simulink model "Simulink_v4"  (R2023b)
settings: Solver=FixedStepDiscrete  StartTime=0.0  StopTime=100  FixedStep=0.01  RelTol=1e-3
settings Model: PacingRate=10  Creator=MrLove  LastModifiedBy=MrLove

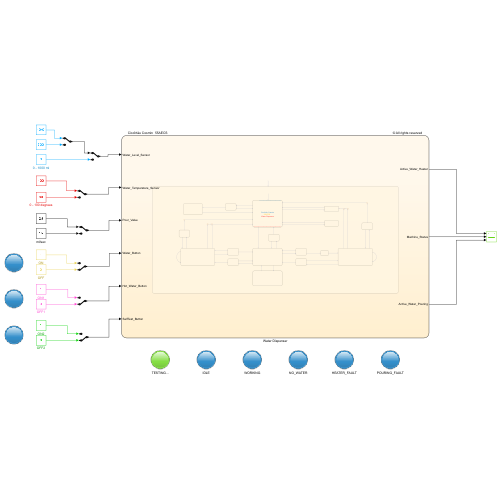
[thumbnail: Simulink's stored preview of the top-level diagram]
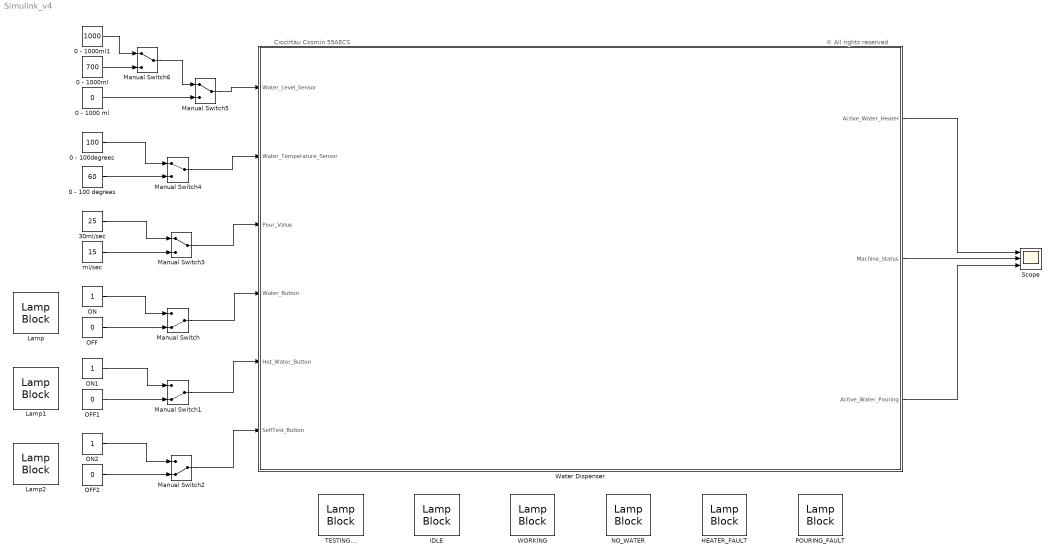
== system Simulink_v4 ==
  note: © All rights reserved
  note: Ciocîrtău Cosmin 55AECS
  0 - 100 degrees : Constant  Value=60
  0 - 1000 ml : Constant  Value=0
  0 - 1000ml : Constant  Value=700
  0 - 1000ml1 : Constant  Value=1000
  0 - 100degrees : Constant  Value=100
  30ml/sec : Constant  Value=25
  HEATER_FAULT : LampBlock  LabelPosition=Hide
  IDLE : LampBlock  LabelPosition=Hide
  Lamp : LampBlock  LabelPosition=Hide
  Lamp1 : LampBlock  LabelPosition=Hide
  Lamp2 : LampBlock  LabelPosition=Hide
  Manual Switch : ManualSwitch  CurrentSetting=0
  Manual Switch1 : ManualSwitch  CurrentSetting=0
  Manual Switch2 : ManualSwitch  CurrentSetting=0
  Manual Switch{3..6} (4 alike) : ManualSwitch
  NO_WATER : LampBlock  LabelPosition=Hide
  OFF : Constant  Value=0  OutDataTypeStr=boolean
  OFF1 : Constant  Value=0  OutDataTypeStr=boolean
  OFF2 : Constant  Value=0
  ON : Constant  OutDataTypeStr=boolean
  ON1 : Constant  OutDataTypeStr=boolean
  ON2 : Constant
  POURING_FAULT : LampBlock  LabelPosition=Hide
  Scope : Scope  NumInputPorts=3
  TESTING... : LampBlock  LabelPosition=Hide
  WORKING : LampBlock  LabelPosition=Hide
  Water Dispenser : Stateflow chart  TreatAsAtomicUnit=on
  ml/sec : Constant  Value=15
  wires:
  Water Dispenser/2(Machine_Status) -> Scope/2
  Water Dispenser/1(Active_Water_Heater) -> Scope/1
  Water Dispenser/3(Active_Water_Pouring) -> Scope/3
  Manual Switch/1 -> Water Dispenser/4(Water_Button)
  ON/1 -> Manual Switch/1
  OFF/1 -> Manual Switch/2
  ON1/1 -> Manual Switch1/1
  OFF1/1 -> Manual Switch1/2
  Manual Switch1/1 -> Water Dispenser/5(Hot_Water_Button)
  ON2/1 -> Manual Switch2/1
  OFF2/1 -> Manual Switch2/2
  Manual Switch2/1 -> Water Dispenser/6(SelfTest_Button)
  30ml/sec/1 -> Manual Switch3/1
  Manual Switch3/1 -> Water Dispenser/3(Pour_Value)
  ml/sec/1 -> Manual Switch3/2
  0 - 100 degrees/1 -> Manual Switch4/2
  0 - 100degrees/1 -> Manual Switch4/1
  Manual Switch4/1 -> Water Dispenser/2(Water_Temperature_Sensor)
  0 - 1000 ml/1 -> Manual Switch5/2
  Manual Switch5/1 -> Water Dispenser/1(Water_Level_Sensor)
  0 - 1000ml/1 -> Manual Switch6/2
  0 - 1000ml1/1 -> Manual Switch6/1
  Manual Switch6/1 -> Manual Switch5/1

== stateflow chart Simulink_v4/Water Dispenser ==
  state WATER_DISPENSER
    note: _______________________
    state SELF_TEST
      en:
      Machine_Status = 5;
      Active_Water_Pouring = Active_Water_Pouring + Pour_Value;
      note: Ciocîrtău Cosmin
          | 55AECS
          | Water Dispenser
      note: _____________________________
    state POURING_FAULT
      en:
      Machine_Status = 4;
    state AFTER_2_SEC
    state NO_WATER
      en:
      Machine_Status = 2;
    state HEATER_FAULT
      en:
      Machine_Status = 3;
    state WAIT_DEBOUCING7
    state WAIT_DEBOUCING6
    state WAIT_DEBOUCING5
    state Cold_Water
      en:
      Active_Water_Pouring = 1;
      Machine_Status = 1;
    state WAIT_DEBOUCING1
    state WAIT
      en:
      Machine_Status = 1;
      Active_Water_Heater = 0;
      Active_Water_Pouring = 0;
    state WAIT_DEBOUCING3
    state Hot_Water
      en:
      Active_Water_Pouring = 1;
      Active_Water_Heater = 0;
      Machine_Status = 1;
    state Wait_500msec
    state WAIT_DEBOUCING4
    state WAIT_DEBOUCING2
    state IDLE
      en:
      Machine_Status = 0;
    (default) -> SELF_TEST : {Active_Water_Heater = 1;
        |  Active_Water_Pouring = 0;
        |  Count = 0;
        |  Count_ml = 0;}
    (junction 107) -> SELF_TEST
    WAIT_DEBOUCING7 -> (junction 107) [order 1] : [after(200,msec)]
        | {Active_Water_Pouring = 0;
        |  Count = 0;}
    SELF_TEST -> AFTER_2_SEC [order 2] : [(after(1, sec)) && (Count < 20)]
    AFTER_2_SEC -> POURING_FAULT [order 1] : [(Active_Water_Pouring < 50 && Count == 1)]
    NO_WATER -> SELF_TEST : [(Water_Level_Sensor > 0) && SelfTest_Button == 1]
        | {Active_Water_Pouring = 0; Count = 0;}
    AFTER_2_SEC -> SELF_TEST [order 2] : {Count = Count + 1;}
    (junction 78) -> NO_WATER
    (junction 141) -> (junction 78)
    Hot_Water -> (junction 78) [order 1] : [Water_Level_Sensor == 0]
        | {Active_Water_Pouring = 0;}
    Hot_Water -> (junction 141) [order 5] : [Count_ml >= Water_Level_Sensor]
    SELF_TEST -> NO_WATER [order 1] : [(Water_Level_Sensor == 0) || Count_ml >= Water_Level_Sensor]
    POURING_FAULT -> SELF_TEST : [SelfTest_Button == 1]{Active_Water_Pouring = 0; Count = 0;}
    (junction 100) -> SELF_TEST
    WAIT_DEBOUCING6 -> (junction 100) [order 1] : [after(200,msec)]
        | {Active_Water_Pouring = 0;
        | Count = 0;}
    HEATER_FAULT -> SELF_TEST : [SelfTest_Button == 1]
        | {Count = 0; Active_Water_Heater = 1;}
    (junction 144) -> (junction 81)
    (junction 81) -> SELF_TEST
    SELF_TEST -> HEATER_FAULT [order 3] : [Water_Temperature_Sensor < 99]{Active_Water_Heater = 0;}
    Cold_Water -> (junction 144) [order 5] : [Count_ml >= Water_Level_Sensor]
        | {Machine_Status = 2;}
    Cold_Water -> (junction 81) [order 1] : [Water_Level_Sensor == 0]
        | {Active_Water_Pouring = 0;
        |  Count = 0;}
    SELF_TEST -> WAIT [order 4] : [Count >= 20]
        | {Active_Water_Pouring = 0;
        |  Active_Water_Heater = 0;}
    WAIT_DEBOUCING5 -> SELF_TEST [order 2] : [after(200,msec)]
        | {Active_Water_Pouring = 0; Count = 0;}
    WAIT_DEBOUCING7 -> Hot_Water [order 2] : [SelfTest_Button == 0]
    Hot_Water -> WAIT_DEBOUCING7 [order 2] : [SelfTest_Button == 1]
    WAIT_DEBOUCING6 -> Cold_Water [order 2] : [SelfTest_Button == 0]
    Cold_Water -> WAIT_DEBOUCING6 [order 2] : [SelfTest_Button == 1]
    WAIT_DEBOUCING5 -> WAIT [order 1] : [SelfTest_Button == 0]
    WAIT -> WAIT_DEBOUCING5 [order 1] : [SelfTest_Button == 1]
    WAIT_DEBOUCING1 -> Cold_Water [order 2] : [Water_Button == 1]
    WAIT_DEBOUCING3 -> WAIT [order 1] : [Hot_Water_Button == 0]
    Cold_Water -> Cold_Water [order 4] : [after(1,sec) && (Count_ml <= Water_Level_Sensor)]
        | {Count_ml = Count_ml + 10;}
    WAIT_DEBOUCING1 -> WAIT [order 1] : [after(200, msec)]
    Hot_Water -> Hot_Water [order 4] : [after(1,sec) && (Count_ml <= Water_Level_Sensor)]
        | {Count_ml = Count_ml + 10;}
    Wait_500msec -> Hot_Water : [after(500, msec)]
    WAIT_DEBOUCING3 -> Wait_500msec [order 2] : [after(200, msec)]
        | {Active_Water_Heater = 1;}
    WAIT -> WAIT_DEBOUCING3 [order 3] : [Hot_Water_Button == 1]
    Cold_Water -> WAIT_DEBOUCING1 [order 3] : [Water_Button == 0]
    WAIT_DEBOUCING4 -> Hot_Water [order 1] : [Hot_Water_Button == 1]
    WAIT_DEBOUCING2 -> WAIT [order 2] : [Water_Button == 0]
    WAIT_DEBOUCING4 -> WAIT [order 2] : [after(200, msec)]
    WAIT_DEBOUCING2 -> Cold_Water [order 1] : [after(200, msec)]
    WAIT -> WAIT_DEBOUCING2 [order 2] : [Water_Button == 1]
    Hot_Water -> WAIT_DEBOUCING4 [order 3] : [Hot_Water_Button == 0]
    IDLE -> WAIT : [Hot_Water_Button == 1 || Water_Button == 1 || SelfTest_Button == 1]
    WAIT -> IDLE [order 4] : [after(120, sec)]
  (default) -> WATER_DISPENSER
  data: Water_Level_Sensor input; Active_Water_Heater output; Machine_Status output; Water_Temperature_Sensor input; Pour_Value input; Active_Water_Pouring output; Water_Button input; Hot_Water_Button input; SelfTest_Button input; Count local; Count_ml local
